simulink model "controle_subespaco"  (R2017a)
settings: Solver=VariableStepAuto  StartTime=0.0  StopTime=10  RelTol=1e-3
values from neighbouring files (symbols this model uses):
  A = [0.976130161834507 0.193278632645524 -0.0437714173532699;-0.181710562635052 0.984060906761371 -0.148925860431169;0.0840316422522322 0.310702671920488 0.699442279329864]    [controle_subespaco.m]    (also in controle_subespaco2.m)
  B = [0.146607054851363;0.251489883468407;0.846034512455990]    [controle_subespaco.m]    (also in controle_subespaco2.m; pseudoInverse.m = inv(A'*A)*A')
  C = Y(i:size(phi*theta,1)+i-1)-(phi*theta)    [MQARX.m]    (also in controle_subespaco.m = [-1.01044391879506 -0.335405568261065 0.249594438654919]; controle_subespaco2.m = [-1.01044391879506 -0.335405568261065 0.249594438654919])
  D = [0.001018347083181]    [controle_subespaco.m]    (also in controle_subespaco2.m)
  k = kb*inv(t)    [controle_subespaco2.m]
  l = inv(t2)*lb'    [controle_subespaco2.m]
settings Model: Creator=Vicente  LastModifiedBy=Vicente

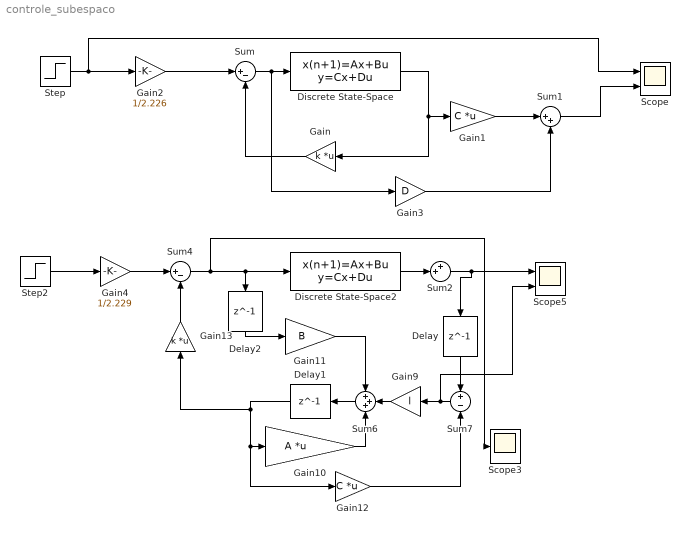
== system controle_subespaco ==
  Delay : Delay  DelayLength=1  InitialCondition=0
  Delay1 : Delay  DelayLength=1  InitialCondition=0
  Delay2 : Delay  DelayLength=1  InitialCondition=0
  Discrete State-Space : DiscreteStateSpace  A=A  B=B  C=eye(3)  D=[0 ;0 ;0]  SampleTime=0.05
  Discrete State-Space2 : DiscreteStateSpace  A=A  B=B  C=C  D=D  SampleTime=0.05
  Gain : Gain  Gain=k  Multiplication=Matrix(K*u)
  Gain1 : Gain  Gain=C  Multiplication=Matrix(K*u)
  Gain10 : Gain  Gain=A  Multiplication=Matrix(K*u)
  Gain11 : Gain  Gain=B
  Gain12 : Gain  Gain=C  Multiplication=Matrix(K*u)
  Gain13 : Gain  Gain=k  Multiplication=Matrix(K*u)
  Gain2 : Gain  Gain=1/2.226
  Gain3 : Gain  Gain=D
  Gain4 : Gain  Gain=1/2.229
  Gain9 : Gain  Gain=l
  Scope : Scope  NumInputPorts=2
  Scope3 : Scope
  Scope5 : Scope  NumInputPorts=2
  Step : Step  Time=4  Before=1  SampleTime=0
  Step2 : Step  Time=4  Before=1  SampleTime=0
  Sum : Sum  Inputs=|+-
  Sum1 : Sum  Inputs=|++
  Sum2 : Sum  Inputs=++|
  Sum4 : Sum  Inputs=|+-
  Sum6 : Sum  Inputs=+++
  Sum7 : Sum  Inputs=+|-
  wires:
  Discrete State-Space/1 -> Gain1/1, Gain/1
  Sum/1 -> Gain3/1, Discrete State-Space/1
  Gain1/1 -> Sum1/1
  Step/1 -> Gain2/1, Scope/1
  Step2/1 -> Gain4/1
  Delay/1 -> Sum7/1
  Gain9/1 -> Sum6/2
  Sum6/1 -> Delay1/1
  Gain10/1 -> Sum6/3
  Delay2/1 -> Gain11/1
  Gain11/1 -> Sum6/1
  Delay1/1 -> Gain13/1, Gain10/1, Gain12/1
  Gain13/1 -> Sum4/2
  Gain12/1 -> Sum7/2
  Sum1/1 -> Scope/2
  Gain3/1 -> Sum1/2
  Sum4/1 -> Scope3/1, Delay2/1, Discrete State-Space2/1
  Gain/1 -> Sum/2
  Gain2/1 -> Sum/1
  Gain4/1 -> Sum4/1
  Discrete State-Space2/1 -> Sum2/2
  Sum2/1 -> Delay/1, Scope5/1
  ? -> Sum2/1
  Sum7/1 -> Scope5/2, Gain9/1
